simulink library "dummyTakeOffToLanding_cl"  (R2020a)
settings: Solver=VariableStepAuto  StartTime=0.0  StopTime=10.0  RelTol=1e-3
undefined symbols (not defined in the file or in its folder): boatSpeed, env, FLIGHTCONTROLLER, fltCtrl, initializeBussesFromBlock, takeoffToLanding, takeoffToLanding_cl, vhcl
libraries: dspsigops x2, periodicCtrlExpStateMachine x1
settings Model: Creator=jcreed2  LastModifiedBy=jcreed2

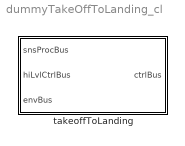
== system dummyTakeOffToLanding_cl ==
  takeoffToLanding : Subsystem  AncestorBlock=takeoffToLanding_cl/takeoffToLanding  LoadFcn=initializeBussesFromBlock(gcb)  InitFcn=initializeBussesFromBlock(gcb)  StartFcn=initializeBussesFromBlock(gcb)  VariantControl=strcmpi(FLIGHTCONTROLLER,'takeoffToLanding')  mask{initPosForInitSStar=vhcl.initPosVecGnd.Value, fluidDensity=env.water.density.Value, pathCtrl=fltCtrl, aeroStruct=vhcl.struct('OCT.aeroSurf')}
      mask prompts: initPosForInitSStar "Initial Position"; fluidDensity "Fluid Density"; pathCtrl "Controller"; aeroStruct "Aerodynamic Structure"
      settings: MinAlgLoopOccurrences=on
      mask DialogControl Container3 Prompt: courseFollow Params
      mask DialogControl Container4 Prompt: setpointToOutput Params

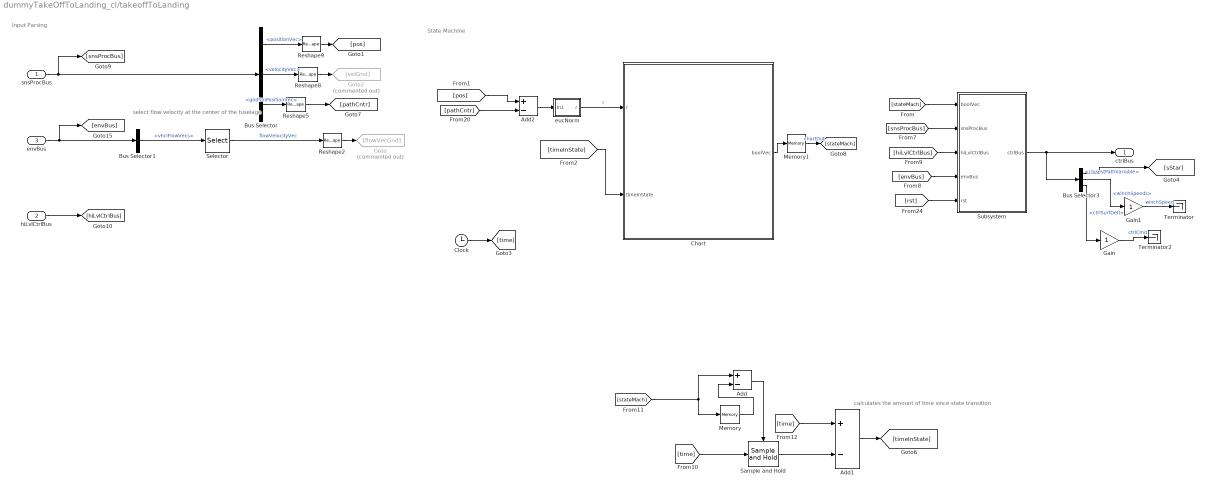
== system dummyTakeOffToLanding_cl/takeoffToLanding ==
  note: calculates the amount of time since state transition
  note: Input Parsing
  note: select flow velocity at the center of the fuselage
  note: State Machine
  snsProcBus : Inport  OutDataTypeStr=Bus: sensorsProcessingBus
  hiLvlCtrlBus : Inport  Port=2  OutDataTypeStr=Bus: hiLvlCtrlBus
  envBus : Inport  Port=3  OutDataTypeStr=Bus: envBus
  Add : Sum  Inputs=+-
  Add1 : Sum  Inputs=+-
  Add2 : Sum  Inputs=+-
  Bus Selector : BusSelector  OutputSignals=positionVec,velocityVec,gndStnPositionVec
  Bus Selector1 : BusSelector  OutputSignals=vhclFlowVecs
  Bus Selector3 : BusSelector  OutputSignals=closestPathVariable,winchSpeeds,ctrlSurfDefl
  Chart : Stateflow chart  TreatAsAtomicUnit=on  mask{gain41=fltCtrl.gain4to1.Value, gain23=fltCtrl.gain2to3.Value, maxR=fltCtrl.maxTL.Value, minTL=fltCtrl.initTL.Value, elvPeak=fltCtrl.elvPeak.Value}
      mask prompts: maxR "max kite position magnitude (r)"; minTL "minimum tether length"; elvPeak "elvation peak for phase 1"
  Clock : Clock
  Gain : Gain
  Gain1 : Gain
  Goto : Goto  Commented=on  GotoTag=flowVecGnd
  Goto2 : Goto  Commented=on  GotoTag=velGnd
  Memory : Memory
  Memory1 : Memory  InitialCondition=[1 0 0 0]
  Reshape{2,5,8..9} (4 alike) : Reshape  OutputDimensionality=Column vector (2-D)
  Sample and Hold : dspsigops/Sample and Hold  trig=Rising edge  initCond=0  latchinput=off
  Selector : Selector  NumberOfDimensions=2  InputPortWidth=3  IndexOptions=Select all,Index vector (dialog)  Indices=[1 3],5  OutputSizes=1,1
  Subsystem : Subsystem
  Terminator : Terminator
  Terminator2 : Terminator
  eucNorm : Subsystem
  ctrlBus : Outport  OutDataTypeStr=Bus: fltCtrlBus  VectorParamsAs1DForOutWhenUnconnected=off
  wires:
  Gain1/1 -> Terminator/1  "winchSpeed"
  Gain/1 -> Terminator2/1  "ctrlCmd"
  Bus Selector3/3 -> Gain/1  "<ctrlSurfDefl>"
  Clock/1 -> [time]
  Bus Selector3/2 -> Gain1/1  "<winchSpeeds>"
  [stateMach] -> Subsystem/1(boolVec)
  [rst] -> Subsystem/5("rst ")
  [envBus] -> Subsystem/4(envBus)
  [hiLvlCtrlBus] -> Subsystem/3(hiLvlCtrlBus)
  [snsProcBus] -> Subsystem/2(snsProcBus)
  Subsystem/1(ctrlBus) -> Bus Selector3/1, ctrlBus/1
  Bus Selector3/1 -> [sStar]  "<closestPathVariable>"
  eucNorm/1(r) -> Chart/1(r)  "r"
  Add2/1 -> eucNorm/1(In1)
  [pathCntr] -> Add2/2
  Bus Selector/3 -> Reshape5/1  "<gndStnPositionVec>"
  Reshape5/1 -> [pathCntr]
  Memory1/1 -> [stateMach]  "chartOut"
  hiLvlCtrlBus/1 -> [hiLvlCtrlBus]
  Chart/1(boolVec) -> Memory1/1
  [pos] -> Add2/1
  Bus Selector1/1 -> Selector/1  "<vhclFlowVecs>"
  envBus/1 -> Bus Selector1/1, [envBus]
  Selector/1 -> Reshape2/1  "flowVelocityVec"
  Reshape9/1 -> [pos]
  Reshape8/1 -> Goto2/1
  Reshape2/1 -> Goto/1
  Bus Selector/1 -> Reshape9/1  "<positionVec>"
  Bus Selector/2 -> Reshape8/1  "<velocityVec>"
  snsProcBus/1 -> Bus Selector/1, [snsProcBus]
  Memory/1 -> Add/2
  Sample and Hold/1 -> Add1/2
  [time] -> Sample and Hold/1
  [stateMach] -> Memory/1, Add/1
  Add/1 -> Sample and Hold/Trigger
  [time] -> Add1/1
  Add1/1 -> [timeInState]
  [timeInState] -> Chart/2(timeInState)

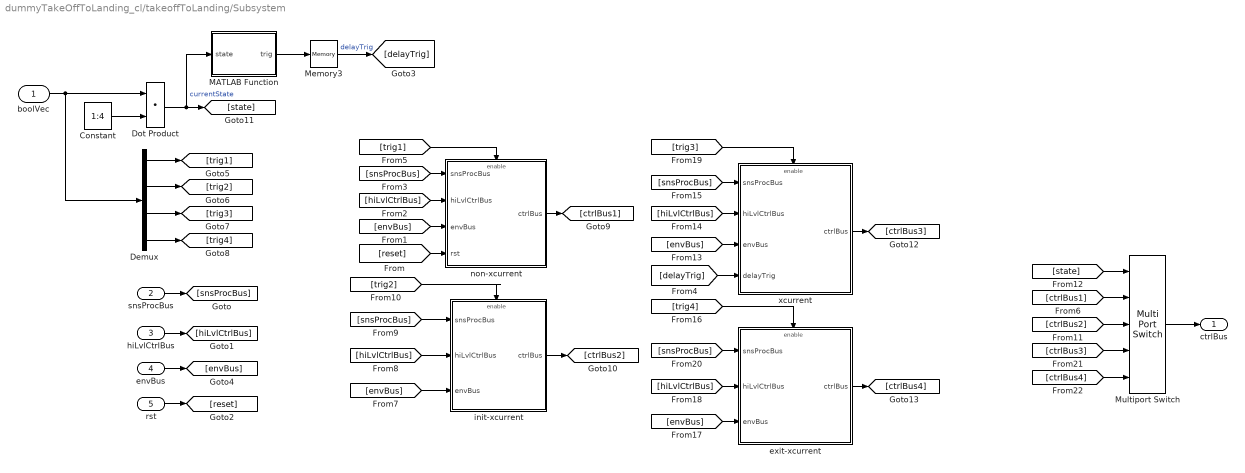
== system dummyTakeOffToLanding_cl/takeoffToLanding/Subsystem ==
  boolVec : Inport
  snsProcBus : Inport  Port=2
  hiLvlCtrlBus : Inport  Port=3
  envBus : Inport  Port=4
  "rst " : Inport  Port=5
  Constant : Constant  Value=1:4
  Demux : Demux
  Dot Product : DotProduct  InputSameDT=on  OutDataTypeStr=Inherit: Inherit via internal rule
  MATLAB Function : MATLAB Function  TreatAsAtomicUnit=on
  Memory3 : Memory
  Multiport Switch : MultiPortSwitch  Inputs=4  DataPortIndices={1,2,3,4,5,6}  DiagnosticForDefault=Warning
  exit-xcurrent : Subsystem  TreatAsAtomicUnit=on
  init-xcurrent : Subsystem  TreatAsAtomicUnit=on
  non-xcurrent : Subsystem  TreatAsAtomicUnit=on
  xcurrent : Subsystem  TreatAsAtomicUnit=on
  ctrlBus : Outport
  wires:
  [ctrlBus4] -> Multiport Switch/5
  [ctrlBus3] -> Multiport Switch/4
  exit-xcurrent/1(ctrlBus) -> [ctrlBus4]
  xcurrent/1(ctrlBus) -> [ctrlBus3]
  [envBus] -> exit-xcurrent/3(envBus)
  [hiLvlCtrlBus] -> exit-xcurrent/2(hiLvlCtrlBus)
  [snsProcBus] -> exit-xcurrent/1(snsProcBus)
  [trig4] -> exit-xcurrent/Enable
  [trig3] -> xcurrent/Enable
  [envBus] -> xcurrent/3(envBus)
  [hiLvlCtrlBus] -> xcurrent/2(hiLvlCtrlBus)
  [snsProcBus] -> xcurrent/1(snsProcBus)
  [state] -> Multiport Switch/1
  [ctrlBus2] -> Multiport Switch/3
  init-xcurrent/1(ctrlBus) -> [ctrlBus2]
  [trig2] -> init-xcurrent/Enable
  [ctrlBus1] -> Multiport Switch/2
  non-xcurrent/1(ctrlBus) -> [ctrlBus1]
  [trig1] -> non-xcurrent/Enable
  Demux/4 -> [trig4]
  Demux/3 -> [trig3]
  Demux/2 -> [trig2]
  Demux/1 -> [trig1]
  [snsProcBus] -> non-xcurrent/1(snsProcBus)
  [hiLvlCtrlBus] -> non-xcurrent/2(hiLvlCtrlBus)
  [envBus] -> non-xcurrent/3(envBus)
  [reset] -> non-xcurrent/4("rst ")
  hiLvlCtrlBus/1 -> [hiLvlCtrlBus]
  "rst "/1 -> [reset]
  envBus/1 -> [envBus]
  snsProcBus/1 -> [snsProcBus]
  [delayTrig] -> xcurrent/4(delayTrig)
  Multiport Switch/1 -> ctrlBus/1
  Memory3/1 -> [delayTrig]  "delayTrig"
  MATLAB Function/1(trig) -> Memory3/1
  Constant/1 -> Dot Product/2
  [envBus] -> init-xcurrent/3(envBus)
  Dot Product/1 -> MATLAB Function/1(state), [state]  "currentState"
  [hiLvlCtrlBus] -> init-xcurrent/2(hiLvlCtrlBus)
  boolVec/1 -> Dot Product/1, Demux/1
  [snsProcBus] -> init-xcurrent/1(snsProcBus)

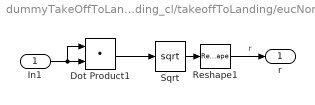
== system dummyTakeOffToLanding_cl/takeoffToLanding/eucNorm ==
  In1 : Inport
  Dot Product1 : DotProduct  InputSameDT=on  OutDataTypeStr=Inherit: Inherit via internal rule
  Reshape1 : Reshape
  Sqrt : Sqrt  SaturateOnIntegerOverflow=on
  r : Outport
  wires:
  Dot Product1/1 -> Sqrt/1
  Reshape1/1 -> r/1  "r"
  In1/1 -> Dot Product1/1, Dot Product1/2
  Sqrt/1 -> Reshape1/1

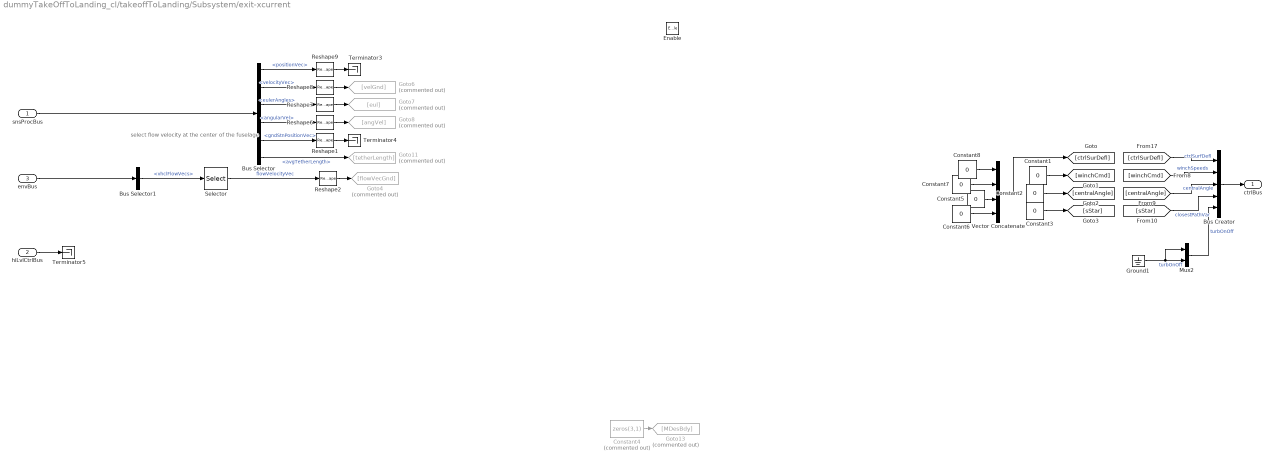
== system dummyTakeOffToLanding_cl/takeoffToLanding/Subsystem/exit-xcurrent ==
  note: select flow velocity at the center of the fuselage
  snsProcBus : Inport  OutDataTypeStr=Bus: sensorsProcessingBus
  hiLvlCtrlBus : Inport  Port=2  OutDataTypeStr=Bus: hiLvlCtrlBus
  envBus : Inport  Port=3  OutDataTypeStr=Bus: envBus
  Enable : EnablePort
  Bus Creator : BusCreator  Inputs=5  OutDataTypeStr=Bus: fltCtrlBus
      settings: InheritFromInputs=off
  Bus Selector : BusSelector  OutputSignals=positionVec,velocityVec,eulerAngles,angularVel,gndStnPositionVec,avgTetherLength
  Bus Selector1 : BusSelector  OutputSignals=vhclFlowVecs
  Constant{1..3,5..8} (7 alike) : Constant  Value=0
  Constant4 : Constant  Commented=on  Value=zeros(3,1)
  Goto11 : Goto  Commented=on  GotoTag=tetherLength
  Goto13 : Goto  Commented=on  GotoTag=MDesBdy
  Goto4 : Goto  Commented=on  GotoTag=flowVecGnd
  Goto6 : Goto  Commented=on  GotoTag=velGnd
  Goto7 : Goto  Commented=on  GotoTag=eul
  Goto8 : Goto  Commented=on  GotoTag=angVel
  Ground1 : Ground
  Mux2 : Mux  Inputs=2
  Reshape{1..2,6..9} (6 alike) : Reshape  OutputDimensionality=Column vector (2-D)
  Selector : Selector  NumberOfDimensions=2  InputPortWidth=3  IndexOptions=Select all,Index vector (dialog)  Indices=[1 3],5  OutputSizes=1,1
  Terminator3 : Terminator
  Terminator4 : Terminator
  Terminator5 : Terminator
  Vector Concatenate : Concatenate  NumInputs=4
  ctrlBus : Outport  OutDataTypeStr=Bus: fltCtrlBus  VectorParamsAs1DForOutWhenUnconnected=off
  wires:
  Ground1/1 -> Mux2/1, Mux2/2  "turbOnOff"
  Mux2/1 -> Bus Creator/5  "turbOnOff"
  Constant7/1 -> Vector Concatenate/2
  Constant8/1 -> Vector Concatenate/1
  Constant6/1 -> Vector Concatenate/4
  Constant5/1 -> Vector Concatenate/3
  hiLvlCtrlBus/1 -> Terminator5/1
  Constant4/1 -> Goto13/1
  Vector Concatenate/1 -> [ctrlSurDefl]
  Bus Selector/6 -> Goto11/1  "<avgTetherLength>"
  Reshape6/1 -> Goto8/1
  snsProcBus/1 -> Bus Selector/1
  Reshape1/1 -> Terminator4/1
  envBus/1 -> Bus Selector1/1
  Bus Selector1/1 -> Selector/1  "<vhclFlowVecs>"
  Reshape2/1 -> Goto4/1
  Bus Selector/5 -> Reshape1/1  "<gndStnPositionVec>"
  Reshape9/1 -> Terminator3/1
  Selector/1 -> Reshape2/1  "flowVelocityVec"
  Reshape8/1 -> Goto6/1
  Bus Selector/4 -> Reshape6/1  "<angularVel>"
  Reshape7/1 -> Goto7/1
  Bus Selector/2 -> Reshape8/1  "<velocityVec>"
  Bus Selector/3 -> Reshape7/1  "<eulerAngles>"
  Bus Selector/1 -> Reshape9/1  "<positionVec>"
  Constant3/1 -> [sStar]
  Constant2/1 -> [centralAngle]
  Constant1/1 -> [winchCmd]
  [centralAngle] -> Bus Creator/3  "centralAngle"
  Bus Creator/1 -> ctrlBus/1
  [winchCmd] -> Bus Creator/2  "winchSpeeds"
  [ctrlSurDefl] -> Bus Creator/1  "ctrlSurfDefl"
  [sStar] -> Bus Creator/4  "closestPathVar"

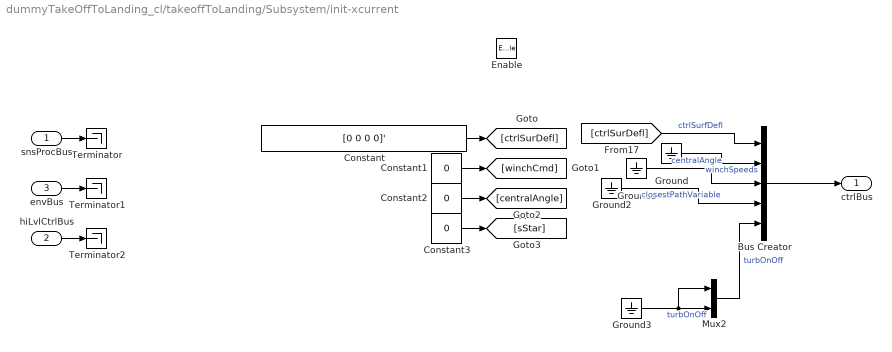
== system dummyTakeOffToLanding_cl/takeoffToLanding/Subsystem/init-xcurrent ==
  snsProcBus : Inport  OutDataTypeStr=Bus: sensorsProcessingBus
  hiLvlCtrlBus : Inport  Port=2  OutDataTypeStr=Bus: hiLvlCtrlBus
  envBus : Inport  Port=3  OutDataTypeStr=Bus: envBus
  Enable : EnablePort
  Bus Creator : BusCreator  Inputs=5  OutDataTypeStr=Bus: fltCtrlBus
      settings: InheritFromInputs=off
  Constant : Constant  Value=[0 0 0 0]'
  Constant1 : Constant  Value=0
  Constant2 : Constant  Value=0
  Constant3 : Constant  Value=0
  Ground{,1..3} (4 alike) : Ground
  Mux2 : Mux  Inputs=2
  Terminator : Terminator
  Terminator1 : Terminator
  Terminator2 : Terminator
  ctrlBus : Outport  OutDataTypeStr=Bus: fltCtrlBus  VectorParamsAs1DForOutWhenUnconnected=off
  wires:
  Mux2/1 -> Bus Creator/5  "turbOnOff"
  Ground3/1 -> Mux2/1, Mux2/2  "turbOnOff"
  Constant/1 -> [ctrlSurDefl]
  Constant3/1 -> [sStar]
  Bus Creator/1 -> ctrlBus/1
  Constant1/1 -> [winchCmd]
  Ground2/1 -> Bus Creator/4  "closestPathVariable"
  snsProcBus/1 -> Terminator/1
  Constant2/1 -> [centralAngle]
  hiLvlCtrlBus/1 -> Terminator2/1
  envBus/1 -> Terminator1/1
  Ground/1 -> Bus Creator/2  "winchSpeeds"
  Ground1/1 -> Bus Creator/3  "centralAngle"
  [ctrlSurDefl] -> Bus Creator/1  "ctrlSurfDefl"

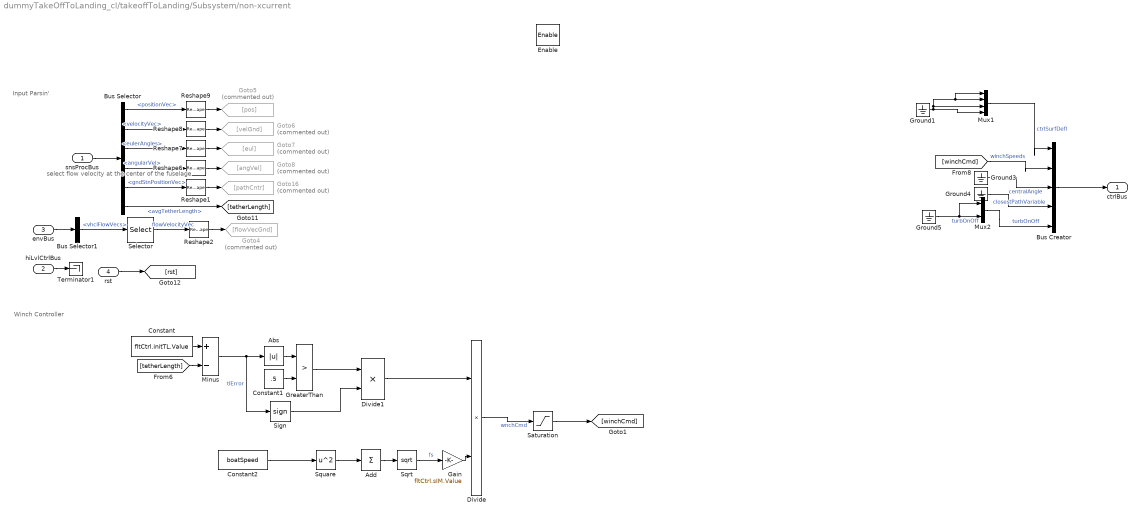
== system dummyTakeOffToLanding_cl/takeoffToLanding/Subsystem/non-xcurrent ==
  note: select flow velocity at the center of the fuselage
  note: Winch Controller
  note: Input Parsin'
  snsProcBus : Inport  OutDataTypeStr=Bus: sensorsProcessingBus
  hiLvlCtrlBus : Inport  Port=2  OutDataTypeStr=Bus: hiLvlCtrlBus
  envBus : Inport  Port=3  OutDataTypeStr=Bus: envBus
  "rst " : Inport  Port=4
  Enable : EnablePort
  Abs : Abs
  Add : Sum  Inputs=+
  Bus Creator : BusCreator  Inputs=5  OutDataTypeStr=Bus: fltCtrlBus
      settings: InheritFromInputs=off
  Bus Selector : BusSelector  OutputSignals=positionVec,velocityVec,eulerAngles,angularVel,gndStnPositionVec,avgTetherLength
  Bus Selector1 : BusSelector  OutputSignals=vhclFlowVecs
  Constant : Constant  Value=fltCtrl.initTL.Value
  Constant1 : Constant  Value=.5
  Constant2 : Constant  Value=boatSpeed
  Divide : Product  Inputs=**
  Divide1 : Product  Inputs=**
  Gain : Gain  Gain=fltCtrl.sIM.Value
  Goto16 : Goto  Commented=on  GotoTag=pathCntr
  Goto4 : Goto  Commented=on  GotoTag=flowVecGnd
  Goto5 : Goto  Commented=on  GotoTag=pos
  Goto6 : Goto  Commented=on  GotoTag=velGnd
  Goto7 : Goto  Commented=on  GotoTag=eul
  Goto8 : Goto  Commented=on  GotoTag=angVel
  GreaterThan : RelationalOperator  Operator=>  OutDataTypeStr=boolean  RndMeth=Simplest
  Ground{1,3..5} (4 alike) : Ground
  Minus : Sum  Inputs=+-
  Mux1 : Mux
  Mux2 : Mux  Inputs=2
  Reshape{1..2,6..9} (6 alike) : Reshape  OutputDimensionality=Column vector (2-D)
  Saturation : Saturate  UpperLimit=0  LowerLimit=-inf
  Selector : Selector  NumberOfDimensions=2  InputPortWidth=3  IndexOptions=Select all,Index vector (dialog)  Indices=[1 3],5  OutputSizes=1,1
  Sign : Signum
  Sqrt : Sqrt  SaturateOnIntegerOverflow=on
  Square : Math  Operator=square  SignedPower=on  SaturateOnIntegerOverflow=on
  Terminator1 : Terminator
  ctrlBus : Outport  OutDataTypeStr=Bus: fltCtrlBus  VectorParamsAs1DForOutWhenUnconnected=off
  wires:
  Ground5/1 -> Mux2/1, Mux2/2  "turbOnOff"
  Mux2/1 -> Bus Creator/5  "turbOnOff"
  Saturation/1 -> [winchCmd]
  GreaterThan/1 -> Divide1/1
  Divide1/1 -> Divide/1
  Sign/1 -> Divide1/2
  Divide/1 -> Saturation/1  "wnchCmd"
  Gain/1 -> Divide/2
  Constant1/1 -> GreaterThan/2
  Abs/1 -> GreaterThan/1
  hiLvlCtrlBus/1 -> Terminator1/1
  "rst "/1 -> [rst]
  Square/1 -> Add/1
  Sqrt/1 -> Gain/1  "fs"
  [tetherLength] -> Minus/2
  Minus/1 -> Abs/1, Sign/1  "tlError"
  Constant/1 -> Minus/1
  Bus Selector/6 -> [tetherLength]  "<avgTetherLength>"
  Add/1 -> Sqrt/1
  Constant2/1 -> Square/1
  Reshape6/1 -> Goto8/1
  snsProcBus/1 -> Bus Selector/1
  Reshape1/1 -> Goto16/1
  envBus/1 -> Bus Selector1/1
  Bus Selector1/1 -> Selector/1  "<vhclFlowVecs>"
  Reshape2/1 -> Goto4/1
  Bus Selector/5 -> Reshape1/1  "<gndStnPositionVec>"
  Reshape9/1 -> Goto5/1
  Selector/1 -> Reshape2/1  "flowVelocityVec"
  Reshape8/1 -> Goto6/1
  Bus Selector/4 -> Reshape6/1  "<angularVel>"
  Reshape7/1 -> Goto7/1
  Bus Selector/2 -> Reshape8/1  "<velocityVec>"
  Bus Selector/3 -> Reshape7/1  "<eulerAngles>"
  Bus Selector/1 -> Reshape9/1  "<positionVec>"
  Ground3/1 -> Bus Creator/3  "centralAngle"
  Bus Creator/1 -> ctrlBus/1
  [winchCmd] -> Bus Creator/2  "winchSpeeds"
  Mux1/1 -> Bus Creator/1  "ctrlSurfDefl"
  Ground4/1 -> Bus Creator/4  "closestPathVariable"
  Ground1/1 -> Mux1/3, Mux1/1, Mux1/2, Mux1/4

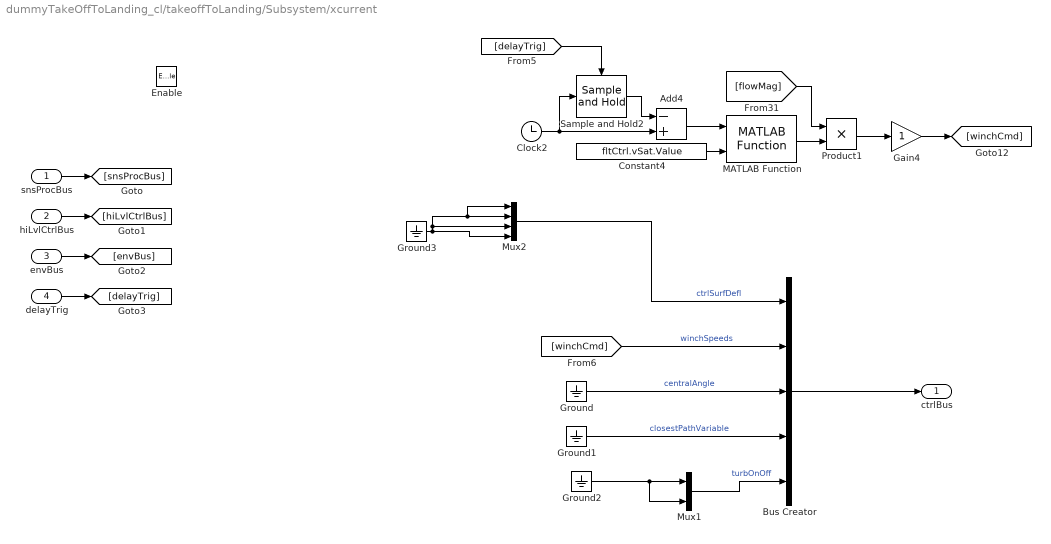
== system dummyTakeOffToLanding_cl/takeoffToLanding/Subsystem/xcurrent ==
  snsProcBus : Inport  OutDataTypeStr=Bus: sensorsProcessingBus
  hiLvlCtrlBus : Inport  Port=2  OutDataTypeStr=Bus: hiLvlCtrlBus
  envBus : Inport  Port=3  OutDataTypeStr=Bus: envBus
  delayTrig : Inport  Port=4
  Enable : EnablePort
  Add4 : Sum  Inputs=-+
  Bus Creator : BusCreator  Inputs=5  OutDataTypeStr=Bus: fltCtrlBus
      settings: InheritFromInputs=off
  Clock2 : Clock
  Constant4 : Constant  Value=fltCtrl.vSat.Value
  Gain4 : Gain
  Ground{,1..3} (4 alike) : Ground
  MATLAB Function : periodicCtrlExpStateMachine/periodicCtrlExpStateMachine/MATLAB Function  SystemSampleTime=-1  Latency=0  AutoFrameSizeCalculation=off
  Mux1 : Mux  Inputs=2
  Mux2 : Mux
  Product1 : Product
  Sample and Hold2 : dspsigops/Sample and Hold  trig=Rising edge  initCond=0  latchinput=off
  ctrlBus : Outport  OutDataTypeStr=Bus: fltCtrlBus  VectorParamsAs1DForOutWhenUnconnected=off
  wires:
  snsProcBus/1 -> [snsProcBus]
  hiLvlCtrlBus/1 -> [hiLvlCtrlBus]
  envBus/1 -> [envBus]
  delayTrig/1 -> [delayTrig]
  Clock2/1 -> Add4/2, Sample and Hold2/1
  Sample and Hold2/1 -> Add4/1
  Constant4/1 -> MATLAB Function/2
  [flowMag] -> Product1/1
  Gain4/1 -> [winchCmd]
  Add4/1 -> MATLAB Function/1
  Product1/1 -> Gain4/1
  MATLAB Function/1 -> Product1/2
  [delayTrig] -> Sample and Hold2/Trigger
  Mux2/1 -> Bus Creator/1  "ctrlSurfDefl"
  Ground1/1 -> Bus Creator/4  "closestPathVariable"
  Ground/1 -> Bus Creator/3  "centralAngle"
  Mux1/1 -> Bus Creator/5  "turbOnOff"
  Ground2/1 -> Mux1/2, Mux1/1
  [winchCmd] -> Bus Creator/2  "winchSpeeds"
  Bus Creator/1 -> ctrlBus/1
  Ground3/1 -> Mux2/3, Mux2/1, Mux2/2, Mux2/4

== matlab function dummyTakeOffToLanding_cl/takeoffToLanding/Subsystem/MATLAB Function ==
  data: state input; trig output
function trig = fcn(state)
trig = 0; 
if state ==3
trig = 1; 
end

== stateflow chart dummyTakeOffToLanding_cl/takeoffToLanding/Chart ==
  state init
    boolVec=[0 1 0 0];
  state non_x
    boolVec=[1 0 0 0];
  state exit
    boolVec=[0 0 0 1];
  state cross
    boolVec=[0 0 1 0];
  (default) -> non_x
  non_x -> init : [r <minTL]
  exit -> non_x : [timeInState>15]
  init -> cross : [timeInState>15]
  cross -> exit : [r > maxR]
  data: boolVec output; r input; timeInState input; maxR parameter; minTL parameter
